simulink model "prepTrajectoryController"  (R2023b)
settings: Solver=VariableStepAuto  StartTime=0.0  StopTime=50  RelTol=1e-3
undefined symbols (not defined in the file): data
libraries: mci_models x2
settings Model: Creator=fluky  LastModifiedBy=fluky

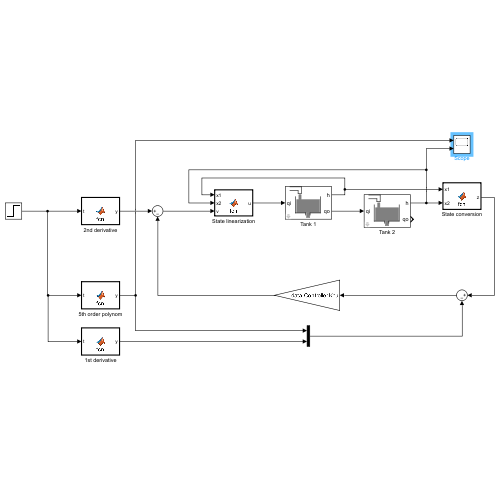
[thumbnail: Simulink's stored preview of the top-level diagram]
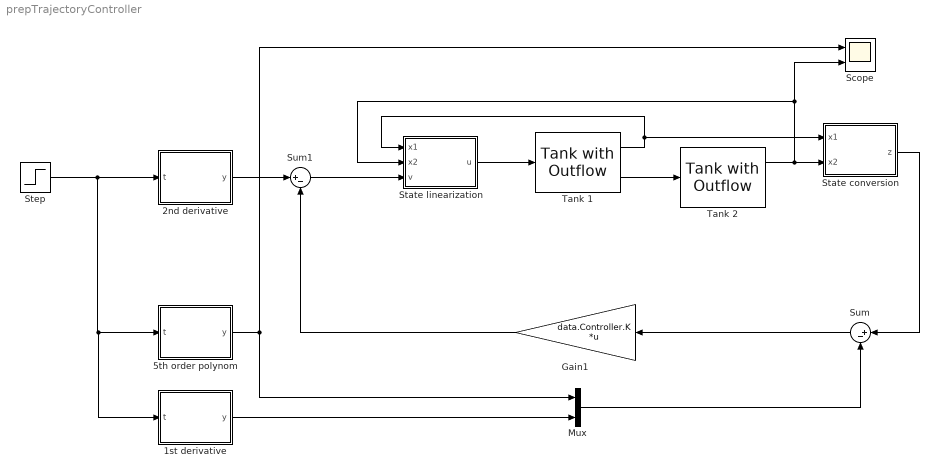
== system prepTrajectoryController ==
  1st derivative : MATLAB Function  TreatAsAtomicUnit=on
  2nd derivative : MATLAB Function  TreatAsAtomicUnit=on
  5th order polynom : MATLAB Function  TreatAsAtomicUnit=on
  Gain1 : Gain  Gain=data.Controller.K  Multiplication=Matrix(K*u)
  Mux : Mux  Inputs=2
  Scope : Scope  NumInputPorts=2
  State conversion : MATLAB Function  TreatAsAtomicUnit=on
  State linearization : MATLAB Function  TreatAsAtomicUnit=on
  Step : Step  After=50  SampleTime=0
  Sum : Sum  Inputs=|+-
  Sum1 : Sum  Inputs=|+-
  Tank 1 : mci_models/Fluid Systems/Tank with Outflow  At=data.At  Ao=data.Aout  rho=data.roh  zeta=data.zeta  g=data.g  h0=data.initHeight
      settings: SourceProductName=MCI Models
  Tank 2 : mci_models/Fluid Systems/Tank with Outflow  At=data.At  Ao=data.Aout  rho=data.roh  zeta=data.zeta  g=data.g  h0=data.initHeight
      settings: SourceProductName=MCI Models
  wires:
  Tank 1/2 -> Tank 2/1
  State linearization/1(u) -> Tank 1/1
  Tank 2/1 -> State linearization/2(x2), Scope/2, State conversion/2(x2)
  State conversion/1(z) -> Sum/1
  Sum/1 -> Gain1/1
  Tank 1/1 -> State conversion/1(x1), State linearization/1(x1)
  Sum1/1 -> State linearization/3(v)
  Gain1/1 -> Sum1/2
  2nd derivative/1(y) -> Sum1/1
  Mux/1 -> Sum/2
  1st derivative/1(y) -> Mux/2
  5th order polynom/1(y) -> Mux/1, Scope/1
  Step/1 -> 1st derivative/1(t), 5th order polynom/1(t), 2nd derivative/1(t)

== matlab function prepTrajectoryController/State conversion ==
  data: x1 input; z output; x2 input; data parameter
function z = fcn(x1, x2, data)

z = [0;0];
z(1) = x2; % is equal to y
z(2) = data.a*sqrt(x1) - data.a*sqrt(x2); % is equal to y_dot

== matlab function prepTrajectoryController/State linearization ==
  data: x1 input; u output; x2 input; v input; data parameter
function u = fcn(x1, x2, v, data)

u = data.roh * data.At * sqrt(x1) * (2*v/data.a + data.a * sqrt(x1/x2));

== matlab function prepTrajectoryController/1st derivative ==
  data: t input; y output; data parameter
function y = fcn(t, data)

if t <= data.traj.T
    y = (data.traj.y2-data.traj.y1)*(6*5*t^4/data.traj.T^5-15*4*t^3/data.traj.T^4+10*3*t^2/data.traj.T^3);
else
    y = 0;
end

== matlab function prepTrajectoryController/5th order polynom ==
  data: t input; y output; data parameter
function y = fcn(t, data)

t = t + 0.0001; % Error otherwise

% Script exp. 5.16
if t <= data.traj.T
    % Trajectory of the system -> smooth at beginning and end
    y = data.traj.y1+(data.traj.y2-data.traj.y1)*(6*(t/data.traj.T)^5-15*(t/data.traj.T)^4+10*(t/data.traj.T)^3);
else
    % End value of the trajectory
    y = data.traj.y2;
end

== matlab function prepTrajectoryController/2nd derivative ==
  data: t input; y output; data parameter
function y = fcn(t, data)

if t <= data.traj.T
    y = (data.traj.y2 - data.traj.y1)*(6*5*4*t^3/data.traj.T^5-15*4*3*t^2/data.traj.T^4+10*3*2*t/data.traj.T^3);
else
    y = 0;
end
